simulink model "Tactical_ACC_trainlm_3_15_Jan_5"  (R2021a)
settings: Solver=FixedStepAuto  StartTime=0.0  StopTime=T  FixedStep=Ts  RelTol=1e-3
undefined symbols (not defined in the file): Ts, v0_ego, v0_lead, x0_ego, x0_lead
libraries: neural x50
(part 2 of 2)

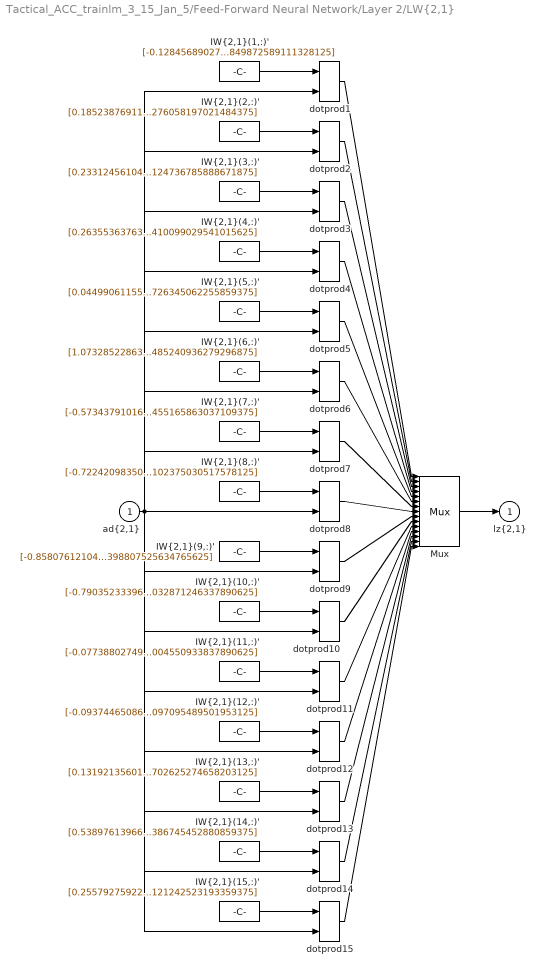
== system Tactical_ACC_trainlm_3_15_Jan_5/Feed-Forward Neural Network/Layer 2/LW{2,1} ==
  "ad{2,1}" : Inport  PortDimensions=15
      mask Display: e = 0.06;c1 = [120 230 180]/255;c2 = ([120 230 180]+0)/(256+128);c3 = ([120 230 180]+128)/(256+128);patch([0 1 1 0],[0 0 1 1],c1);patch([0 1 1 1-e 1-e 0+e],[0 0 1 1-e 0+e 0+e],c2);patch([0 0 1 1-e 0+e 0+e],[0 1 1 1-e 1-e 0+e],c3);plot([0 1 1 0 0],[0 0 1 1 0]);
  "IW{2,1}(1,:)'" : Constant  Value=[-0.1284568902708948245905418161783018149435520172119140625;0.54389311937212003744690491657820530235767364501953125;0.53673915075766809312796112862997688353061676025390625;-0.96084475289336257475270031136460602283477783203125;-0.39150449404426834743020435780636034905910491943359375;-0.1860903257221864226522711760480888187885284423828125;0.7272658289096070038937114077270962297916412353515625;-0.54431412858791627940036050858907401561737060546875;0.5380581706717924017624454791075550019741058349609375;-0.9009348419158775822523921306128613650798797607421875;-0.402444399393438401180134178503067232668399810791015625;-0.5338710106559780843582529996638186275959014892578125;-0.83906258199989902646365180771681480109691619873046875;-0.64876603531735022034609983165864832699298858642578125;0.179996379296625708121837305952794849872589111328125]
      mask Display: e = 0.06;c1 = [120 150 230]/255;c2 = ([120 150 230]+0)/383;c3 = ([120 150 230]+128)/383;patch([0 1 1 0],[0 0 1 1],c1);patch([0 1 1 1-e 1-e 0+e],[0 0 1 1-e 0+e 0+e],c2);patch([0 0 1 1-e 0+e 0+e],[0 1 1 1-e 1-e 0+e],c3);plot([0 1 1 0 0],[0 0 1 1 0]);disp('weights');
  "IW{2,1}(10,:)'" : Constant  Value=[-0.79035233396170545550063479822711087763309478759765625;0.72237775299588691257923755983938463032245635986328125;-0.306611429735239748861630459941807202994823455810546875;0.5382287747765912566677570794126950204372406005859375;0.99699154938168776940443649436929263174533843994140625;0.3573046096003764660054002888500690460205078125;0.59913861015160729817097262639435939490795135498046875;-0.8330343727947546739187600906006991863250732421875;-0.581189831958130564970588238793425261974334716796875;-0.4362662882391401542037101535242982208728790283203125;-0.382792034697409022658831645458121784031391143798828125;1.4688049411392551935051642431062646210193634033203125;0.79640769268750644105381297777057625353336334228515625;-0.4162072596359613907424090939457528293132781982421875;-0.181387517948383314436711089001619257032871246337890625]
      mask Display: e = 0.06;c1 = [120 150 230]/255;c2 = ([120 150 230]+0)/383;c3 = ([120 150 230]+128)/383;patch([0 1 1 0],[0 0 1 1],c1);patch([0 1 1 1-e 1-e 0+e],[0 0 1 1-e 0+e 0+e],c2);patch([0 0 1 1-e 0+e 0+e],[0 1 1 1-e 1-e 0+e],c3);plot([0 1 1 0 0],[0 0 1 1 0]);disp('weights');
  "IW{2,1}(11,:)'" : Constant  Value=[-0.07738802749405981895591821739799343049526214599609375;-0.030300753448414353974360579968561069108545780181884765625;0.13159391893646643634241399922757409512996673583984375;-0.2064169659727668193482941205729730427265167236328125;0.042509571957955911980509000613892567344009876251220703125;-0.0096459618206787833827320355339907109737396240234375;0.374231149766926451949444754063733853399753570556640625;0.25191957034316647678906520013697445392608642578125;0.1045826830775500315695580866304226219654083251953125;0.07719335609068078696282100281678140163421630859375;0.635756796826290493385158697492443025112152099609375;0.10699981116102953715429890735322260297834873199462890625;-0.152211268792612097744409993538283742964267730712890625;-0.164472335625503174316719423586619086563587188720703125;0.79116563379986681869837639169418253004550933837890625]
      mask Display: e = 0.06;c1 = [120 150 230]/255;c2 = ([120 150 230]+0)/383;c3 = ([120 150 230]+128)/383;patch([0 1 1 0],[0 0 1 1],c1);patch([0 1 1 1-e 1-e 0+e],[0 0 1 1-e 0+e 0+e],c2);patch([0 0 1 1-e 0+e 0+e],[0 1 1 1-e 1-e 0+e],c3);plot([0 1 1 0 0],[0 0 1 1 0]);disp('weights');
  "IW{2,1}(12,:)'" : Constant  Value=[-0.09374465086869930574575704440576373599469661712646484375;-0.21310105235882270680036754129105247557163238525390625;-0.10868460812037449014777479305848828516900539398193359375;0.617028191774690260018587650847621262073516845703125;0.77303193361052124910060001639067195355892181396484375;-0.6205791879648396847102276296936906874179840087890625;0.92080509229272256011000763464835472404956817626953125;0.32188911589468460761054302565753459930419921875;0.25976677012884241690926501178182661533355712890625;0.390326078888663996480090645491145551204681396484375;-0.6818652671110874141646718271658755838871002197265625;0.8765389199457593871755989312077872455120086669921875;0.85347912612335619098047345687518827617168426513671875;-0.057448392693464189751040294140693731606006622314453125;-0.7914071094984909127134642403689213097095489501953125]
      mask Display: e = 0.06;c1 = [120 150 230]/255;c2 = ([120 150 230]+0)/383;c3 = ([120 150 230]+128)/383;patch([0 1 1 0],[0 0 1 1],c1);patch([0 1 1 1-e 1-e 0+e],[0 0 1 1-e 0+e 0+e],c2);patch([0 0 1 1-e 0+e 0+e],[0 1 1 1-e 1-e 0+e],c3);plot([0 1 1 0 0],[0 0 1 1 0]);disp('weights');
  "IW{2,1}(13,:)'" : Constant  Value=[0.1319213560109291638600126361779985018074512481689453125;0.342914070048148500458040643934509716928005218505859375;0.17346245905404111820047319270088337361812591552734375;0.5101541980141670595827463330351747572422027587890625;0.2116092910741979860045347550112637691199779510498046875;-0.0099883500195583341252358877682127058506011962890625;0.07323493448403718686368080170723260380327701568603515625;0.459503710634442175120284446165896952152252197265625;-0.9360179684748661799176261411048471927642822265625;-0.0017679730348210132007125139352865517139434814453125;-0.78093606800248605015468683632207103073596954345703125;-0.165663696750330158291575344264856539666652679443359375;-0.26863726210748828382435249295667745172977447509765625;0.443776146337074350878282302801380865275859832763671875;0.475654128018537403210785896590095944702625274658203125]
      mask Display: e = 0.06;c1 = [120 150 230]/255;c2 = ([120 150 230]+0)/383;c3 = ([120 150 230]+128)/383;patch([0 1 1 0],[0 0 1 1],c1);patch([0 1 1 1-e 1-e 0+e],[0 0 1 1-e 0+e 0+e],c2);patch([0 0 1 1-e 0+e 0+e],[0 1 1 1-e 1-e 0+e],c3);plot([0 1 1 0 0],[0 0 1 1 0]);disp('weights');
  "IW{2,1}(14,:)'" : Constant  Value=[0.5389761396637500201478587769088335335254669189453125;0.48251476910261115182976254800450988113880157470703125;0.57826646044851981454115730230114422738552093505859375;-0.2452089103297943051273932724143378436565399169921875;-1.179601056993847318921098121791146695613861083984375;-0.7047835560466226834108738330542109906673431396484375;-0.1688329075373741494647816807628259994089603424072265625;0.78150423265064450362160641816444694995880126953125;0.2294268382342810053131643144297413527965545654296875;0.071602111502226506445367704145610332489013671875;-0.5583507712921489396507013225345872342586517333984375;-1.040588019370590533441145453252829611301422119140625;-0.417402993887157902630491435047588311135768890380859375;0.6362951341913660741056446568109095096588134765625;0.837706070944830738511654999456368386745452880859375]
      mask Display: e = 0.06;c1 = [120 150 230]/255;c2 = ([120 150 230]+0)/383;c3 = ([120 150 230]+128)/383;patch([0 1 1 0],[0 0 1 1],c1);patch([0 1 1 1-e 1-e 0+e],[0 0 1 1-e 0+e 0+e],c2);patch([0 0 1 1-e 0+e 0+e],[0 1 1 1-e 1-e 0+e],c3);plot([0 1 1 0 0],[0 0 1 1 0]);disp('weights');
  "IW{2,1}(15,:)'" : Constant  Value=[0.25579275922833755174679026822559535503387451171875;0.040104934780773593416824951418675482273101806640625;-0.11538917323325836861158677493222057819366455078125;-0.56796216807721133790209933067671954631805419921875;-0.6002743542850959013179590328945778310298919677734375;-0.890051706187623636878925026394426822662353515625;0.6026952110439045551260051070130430161952972412109375;0.964606445767212772324228353681974112987518310546875;-0.2751770754538946928136056158109568059444427490234375;-0.10963366940791541281896570581011474132537841796875;-0.667079118247158486809667010675184428691864013671875;-0.2028210065283138074931912342435680329799652099609375;-0.891521031117740836435814344440586864948272705078125;-0.799556919609016869543438588152639567852020263671875;0.12372285056327481100879595032893121242523193359375]
      mask Display: e = 0.06;c1 = [120 150 230]/255;c2 = ([120 150 230]+0)/383;c3 = ([120 150 230]+128)/383;patch([0 1 1 0],[0 0 1 1],c1);patch([0 1 1 1-e 1-e 0+e],[0 0 1 1-e 0+e 0+e],c2);patch([0 0 1 1-e 0+e 0+e],[0 1 1 1-e 1-e 0+e],c3);plot([0 1 1 0 0],[0 0 1 1 0]);disp('weights');
  "IW{2,1}(2,:)'" : Constant  Value=[0.185238769116202905973267434092122130095958709716796875;0.86572745162572328769812202153843827545642852783203125;-0.5993331590168649025684999287477694451808929443359375;-0.3382842395718579364682909726980142295360565185546875;0.92854655533397656430594224730157293379306793212890625;0.4974114364313828584585053249611519277095794677734375;0.08349591760344533819537815588773810304701328277587890625;-0.003811417607220590753058786503970623016357421875;0.162892975750795532263737186440266668796539306640625;-0.0208600216453564968333012075163424015045166015625;0.09994084869043064200955228670864016748964786529541015625;0.6505716295410695071410600576200522482395172119140625;-0.74344937140645417361639601949718780815601348876953125;0.311377290880280488405418282127357088029384613037109375;-0.370413344649913101047644659047364257276058197021484375]
      mask Display: e = 0.06;c1 = [120 150 230]/255;c2 = ([120 150 230]+0)/383;c3 = ([120 150 230]+128)/383;patch([0 1 1 0],[0 0 1 1],c1);patch([0 1 1 1-e 1-e 0+e],[0 0 1 1-e 0+e 0+e],c2);patch([0 0 1 1-e 0+e 0+e],[0 1 1 1-e 1-e 0+e],c3);plot([0 1 1 0 0],[0 0 1 1 0]);disp('weights');
  "IW{2,1}(3,:)'" : Constant  Value=[0.2331245610411065982692235820650239475071430206298828125;0.94534056286266598956302686929120682179927825927734375;0.73477219805281890341319694925914518535137176513671875;-0.1513810063337250877424366990453563630580902099609375;-1.2712555974780930245771060072002001106739044189453125;0.6511676315723111674316214703139849007129669189453125;0.8116798971944201301909060930483974516391754150390625;0.801704977064009671750000052270479500293731689453125;0.856626124628375951175485170097090303897857666015625;-0.6149792078758504754176783535513095557689666748046875;0.9912444394374702039129942932049743831157684326171875;-1.6174591172065169164540066049084998667240142822265625;0.7343427724308513315776281160651706159114837646484375;-0.373115221066490587720210214683902449905872344970703125;-0.307431976628442071852731487524579279124736785888671875]
      mask Display: e = 0.06;c1 = [120 150 230]/255;c2 = ([120 150 230]+0)/383;c3 = ([120 150 230]+128)/383;patch([0 1 1 0],[0 0 1 1],c1);patch([0 1 1 1-e 1-e 0+e],[0 0 1 1-e 0+e 0+e],c2);patch([0 0 1 1-e 0+e 0+e],[0 1 1 1-e 1-e 0+e],c3);plot([0 1 1 0 0],[0 0 1 1 0]);disp('weights');
  "IW{2,1}(4,:)'" : Constant  Value=[0.26355363763175121416537649565725587308406829833984375;-0.6159994507456831858149826075532473623752593994140625;-0.309763994465098335684416497315396554768085479736328125;-0.4594591531358693803355208729044534265995025634765625;0.366643413083722002898667824410949833691120147705078125;0.579926059889061651375641304184682667255401611328125;0.496490583582257893890954392190906219184398651123046875;0.1493224382603752786735640256665647029876708984375;0.1601807315168832790419628508971072733402252197265625;-0.753832504908109601871046834276057779788970947265625;0.66482363338864047808129953409661538898944854736328125;0.7047628961209226883255496431956999003887176513671875;-0.597867900421577669334283200441859662532806396484375;0.84600607163113539233023630004026927053928375244140625;0.1183481655249266906171357049970538355410099029541015625]
      mask Display: e = 0.06;c1 = [120 150 230]/255;c2 = ([120 150 230]+0)/383;c3 = ([120 150 230]+128)/383;patch([0 1 1 0],[0 0 1 1],c1);patch([0 1 1 1-e 1-e 0+e],[0 0 1 1-e 0+e 0+e],c2);patch([0 0 1 1-e 0+e 0+e],[0 1 1 1-e 1-e 0+e],c3);plot([0 1 1 0 0],[0 0 1 1 0]);disp('weights');
  "IW{2,1}(5,:)'" : Constant  Value=[0.0449906115542042517319032413070090115070343017578125;-0.7222515943416893957618185595492832362651824951171875;-0.9110918154435230231769082820392213761806488037109375;-0.6058924038090884867102658972726203501224517822265625;-0.122710034826088776327424056944437325000762939453125;-0.3629515092020156874497160970349796116352081298828125;0.165581930351680117752266596653498709201812744140625;0.6903563701080732695203323601162992417812347412109375;-0.96603412332547744512112330994568765163421630859375;-0.5890116581846402965538800344802439212799072265625;-0.45941133541460477118789640371687710285186767578125;0.457323363356542333946208600536920130252838134765625;-0.408932331049287167701322687207721173763275146484375;-0.763689603106578740465693044825457036495208740234375;-0.3283020506461509224749306667945347726345062255859375]
      mask Display: e = 0.06;c1 = [120 150 230]/255;c2 = ([120 150 230]+0)/383;c3 = ([120 150 230]+128)/383;patch([0 1 1 0],[0 0 1 1],c1);patch([0 1 1 1-e 1-e 0+e],[0 0 1 1-e 0+e 0+e],c2);patch([0 0 1 1-e 0+e 0+e],[0 1 1 1-e 1-e 0+e],c3);plot([0 1 1 0 0],[0 0 1 1 0]);disp('weights');
  "IW{2,1}(6,:)'" : Constant  Value=[1.073285228639864641309031867422163486480712890625;0.392495340995861308197589778501424007117748260498046875;0.4850650961144948869474546881974674761295318603515625;0.6434423699226197168599128417554311454296112060546875;0.680041364342549581323282836819998919963836669921875;0.0681282547414527872575717992731370031833648681640625;0.64862678540349472111614659297629259526729583740234375;0.47728058399080364182509583770297467708587646484375;-0.7582808578028836787865429869270883500576019287109375;-0.7069701787702202810947937905439175665378570556640625;-0.6662159570437304889622964765294454991817474365234375;0.1711366707004692566673753617578768171370029449462890625;-0.346231314906966514133301870970171876251697540283203125;0.9654623989469779399286153420689515769481658935546875;-0.60325600334875761898700829988229088485240936279296875]
      mask Display: e = 0.06;c1 = [120 150 230]/255;c2 = ([120 150 230]+0)/383;c3 = ([120 150 230]+128)/383;patch([0 1 1 0],[0 0 1 1],c1);patch([0 1 1 1-e 1-e 0+e],[0 0 1 1-e 0+e 0+e],c2);patch([0 0 1 1-e 0+e 0+e],[0 1 1 1-e 1-e 0+e],c3);plot([0 1 1 0 0],[0 0 1 1 0]);disp('weights');
  "IW{2,1}(7,:)'" : Constant  Value=[-0.57343791016769840584998974009067751467227935791015625;-0.81230175846522756355483352308510802686214447021484375;-0.460163965563413768222744693048298358917236328125;-0.140157181233467209580112466937862336635589599609375;0.595545978896323102702581309131346642971038818359375;-0.82009864245883790090374532155692577362060546875;0.7869613238475354766165992259630002081394195556640625;0.17197407165295164332974309218116104602813720703125;0.725421437399339286145050209597684442996978759765625;-0.621855651054772362584799338947050273418426513671875;0.129854351950570212625990507149253971874713897705078125;-0.85541353023072674854887509354739449918270111083984375;-0.066954344696821710414269546163268387317657470703125;0.08686990560648304160462629397443379275500774383544921875;-0.56968257593998483656605458236299455165863037109375]
      mask Display: e = 0.06;c1 = [120 150 230]/255;c2 = ([120 150 230]+0)/383;c3 = ([120 150 230]+128)/383;patch([0 1 1 0],[0 0 1 1],c1);patch([0 1 1 1-e 1-e 0+e],[0 0 1 1-e 0+e 0+e],c2);patch([0 0 1 1-e 0+e 0+e],[0 1 1 1-e 1-e 0+e],c3);plot([0 1 1 0 0],[0 0 1 1 0]);disp('weights');
  "IW{2,1}(8,:)'" : Constant  Value=[-0.7224209835068311491568238125182688236236572265625;0.050869593250156990016375146979044075123965740203857421875;0.21859062205123958033681219603749923408031463623046875;0.7755419085127075451424616403528489172458648681640625;-0.98730531091106688013070424858597107231616973876953125;-0.776588511613593102111963162315078079700469970703125;0.792481707072821617288127526990137994289398193359375;-0.5065309480280502096860573146841488778591156005859375;-0.031406977575795025359184364788234233856201171875;-0.9146951781777132861606105507235042750835418701171875;0.49203673068935105394672291367896832525730133056640625;0.41480058077774961677874898668960668146610260009765625;0.183304582750635047805332078496576286852359771728515625;0.385143116164009813306989826742210425436496734619140625;1.1302421062639844695496549320523627102375030517578125]
      mask Display: e = 0.06;c1 = [120 150 230]/255;c2 = ([120 150 230]+0)/383;c3 = ([120 150 230]+128)/383;patch([0 1 1 0],[0 0 1 1],c1);patch([0 1 1 1-e 1-e 0+e],[0 0 1 1-e 0+e 0+e],c2);patch([0 0 1 1-e 0+e 0+e],[0 1 1 1-e 1-e 0+e],c3);plot([0 1 1 0 0],[0 0 1 1 0]);disp('weights');
  "IW{2,1}(9,:)'" : Constant  Value=[-0.85807612104994845925176605305750854313373565673828125;0.060642466524505611591422393757966347038745880126953125;0.67053556318306017924868456248077563941478729248046875;-0.2176340090776733848798585313488729298114776611328125;0.498101819152965752390826992268557660281658172607421875;-0.727414902123402651312744637834839522838592529296875;-1.0967891667210161177337113258545286953449249267578125;0.3328324346389359700282284393324516713619232177734375;0.6897113491525264095116654061712324619293212890625;0.270395833719764056013445951975882053375244140625;-0.1297060102155986049954350391999469138681888580322265625;0.62727037435593546721435131985344924032688140869140625;-0.9040101576978389896765975208836607635021209716796875;1.003263748472904115516257661511190235614776611328125;0.541537544987497287962696645990945398807525634765625]
      mask Display: e = 0.06;c1 = [120 150 230]/255;c2 = ([120 150 230]+0)/383;c3 = ([120 150 230]+128)/383;patch([0 1 1 0],[0 0 1 1],c1);patch([0 1 1 1-e 1-e 0+e],[0 0 1 1-e 0+e 0+e],c2);patch([0 0 1 1-e 0+e 0+e],[0 1 1 1-e 1-e 0+e],c3);plot([0 1 1 0 0],[0 0 1 1 0]);disp('weights');
  Mux : Mux  Inputs=15
      mask Display: e = 0.06;c1 = [120 150 230]/255;c2 = ([120 150 230]+0)/383;c3 = ([120 150 230]+128)/383;patch([0 1 1 0],[0 0 1 1],c1);patch([0 1 1 1-e 1-e 0+e],[0 0 1 1-e 0+e 0+e],c2);patch([0 0 1 1-e 0+e 0+e],[0 1 1 1-e 1-e 0+e],c3);plot([0 1 1 0 0],[0 0 1 1 0]);disp('Mux');
  dotprod{1..15} (15 alike) : neural/Weight Functions/dotprod
  "lz{2,1}" : Outport
      mask Display: e = 0.06;c1 = [120 230 180]/255;c2 = ([120 230 180]+0)/(256+128);c3 = ([120 230 180]+128)/(256+128);patch([0 1 1 0],[0 0 1 1],c1);patch([0 1 1 1-e 1-e 0+e],[0 0 1 1-e 0+e 0+e],c2);patch([0 0 1 1-e 0+e 0+e],[0 1 1 1-e 1-e 0+e],c3);plot([0 1 1 0 0],[0 0 1 1 0]);
  wires:
  "IW{2,1}(1,:)'"/1 -> dotprod1/1
  "ad{2,1}"/1 -> dotprod1/2, dotprod2/2, dotprod3/2, dotprod4/2, dotprod5/2, dotprod6/2, dotprod7/2, dotprod8/2, dotprod9/2, dotprod10/2, dotprod11/2, dotprod12/2, dotprod13/2, dotprod14/2, dotprod15/2
  dotprod1/1 -> Mux/1
  "IW{2,1}(2,:)'"/1 -> dotprod2/1
  dotprod2/1 -> Mux/2
  "IW{2,1}(3,:)'"/1 -> dotprod3/1
  dotprod3/1 -> Mux/3
  "IW{2,1}(4,:)'"/1 -> dotprod4/1
  dotprod4/1 -> Mux/4
  "IW{2,1}(5,:)'"/1 -> dotprod5/1
  dotprod5/1 -> Mux/5
  "IW{2,1}(6,:)'"/1 -> dotprod6/1
  dotprod6/1 -> Mux/6
  "IW{2,1}(7,:)'"/1 -> dotprod7/1
  dotprod7/1 -> Mux/7
  "IW{2,1}(8,:)'"/1 -> dotprod8/1
  dotprod8/1 -> Mux/8
  "IW{2,1}(9,:)'"/1 -> dotprod9/1
  dotprod9/1 -> Mux/9
  "IW{2,1}(10,:)'"/1 -> dotprod10/1
  dotprod10/1 -> Mux/10
  "IW{2,1}(11,:)'"/1 -> dotprod11/1
  dotprod11/1 -> Mux/11
  "IW{2,1}(12,:)'"/1 -> dotprod12/1
  dotprod12/1 -> Mux/12
  "IW{2,1}(13,:)'"/1 -> dotprod13/1
  dotprod13/1 -> Mux/13
  "IW{2,1}(14,:)'"/1 -> dotprod14/1
  dotprod14/1 -> Mux/14
  "IW{2,1}(15,:)'"/1 -> dotprod15/1
  dotprod15/1 -> Mux/15
  Mux/1 -> "lz{2,1}"/1

== system Tactical_ACC_trainlm_3_15_Jan_5/Feed-Forward Neural Network/Layer 3/Delays 1 ==
  "p{3}" : Inport  PortDimensions=15
      mask Display: e = 0.06;c1 = [120 230 180]/255;c2 = ([120 230 180]+0)/(256+128);c3 = ([120 230 180]+128)/(256+128);patch([0 1 1 0],[0 0 1 1],c1);patch([0 1 1 1-e 1-e 0+e],[0 0 1 1-e 0+e 0+e],c2);patch([0 0 1 1-e 0+e 0+e],[0 1 1 1-e 1-e 0+e],c3);plot([0 1 1 0 0],[0 0 1 1 0]);
  mux : Mux  Inputs=1
      mask Display: e = 0.06;c1 = [120 150 230]/255;c2 = ([120 150 230]+0)/383;c3 = ([120 150 230]+128)/383;patch([0 1 1 0],[0 0 1 1],c1);patch([0 1 1 1-e 1-e 0+e],[0 0 1 1-e 0+e 0+e],c2);patch([0 0 1 1-e 0+e 0+e],[0 1 1 1-e 1-e 0+e],c3);plot([0 1 1 0 0],[0 0 1 1 0]);disp('Mux')
  "pd{3,2}" : Outport
      mask Display: e = 0.06;c1 = [120 230 180]/255;c2 = ([120 230 180]+0)/(256+128);c3 = ([120 230 180]+128)/(256+128);patch([0 1 1 0],[0 0 1 1],c1);patch([0 1 1 1-e 1-e 0+e],[0 0 1 1-e 0+e 0+e],c2);patch([0 0 1 1-e 0+e 0+e],[0 1 1 1-e 1-e 0+e],c3);plot([0 1 1 0 0],[0 0 1 1 0]);
  wires:
  "p{3}"/1 -> mux/1
  mux/1 -> "pd{3,2}"/1

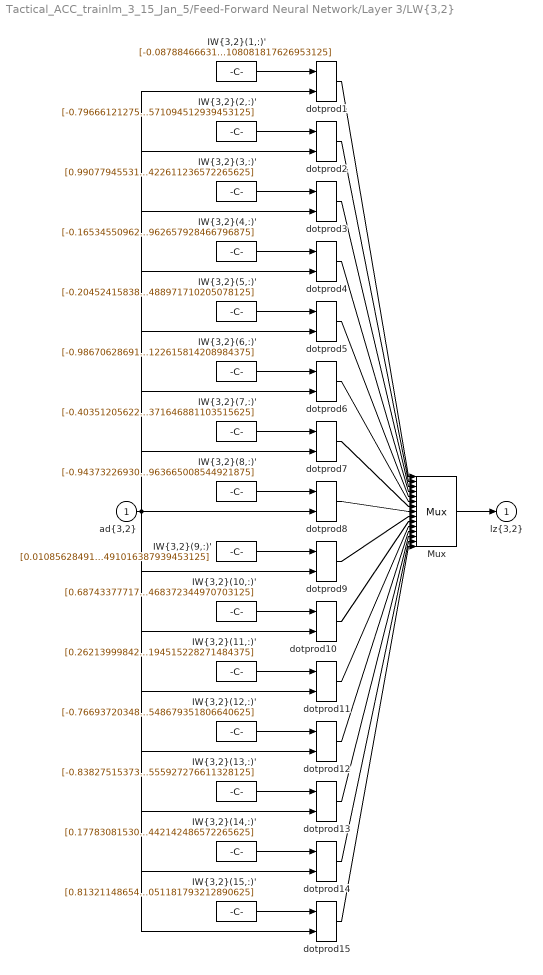
== system Tactical_ACC_trainlm_3_15_Jan_5/Feed-Forward Neural Network/Layer 3/LW{3,2} ==
  "ad{3,2}" : Inport  PortDimensions=15
      mask Display: e = 0.06;c1 = [120 230 180]/255;c2 = ([120 230 180]+0)/(256+128);c3 = ([120 230 180]+128)/(256+128);patch([0 1 1 0],[0 0 1 1],c1);patch([0 1 1 1-e 1-e 0+e],[0 0 1 1-e 0+e 0+e],c2);patch([0 0 1 1-e 0+e 0+e],[0 1 1 1-e 1-e 0+e],c3);plot([0 1 1 0 0],[0 0 1 1 0]);
  "IW{3,2}(1,:)'" : Constant  Value=[-0.0878846663125170124430951545946300029754638671875;0.0675439035340004156893201070488430559635162353515625;0.3850639727730376105085952076478861272335052490234375;-0.897336227775257899708094555535353720188140869140625;0.4800646559755552544856982422061264514923095703125;-0.5886509570704803184781894742627628147602081298828125;-0.7754320756879466980393544872640632092952728271484375;-0.0247924491321527273868241536547429859638214111328125;-0.81529532256159686909313677460886538028717041015625;-0.367142001707418064171406513196416199207305908203125;0.9758694699049907939070180873386561870574951171875;-0.2984465102282147785928145822254009544849395751953125;-0.750254482560374302835271009826101362705230712890625;-0.07347884281256167327001094236038625240325927734375;0.61840770258758670507859278586693108081817626953125]
      mask Display: e = 0.06;c1 = [120 150 230]/255;c2 = ([120 150 230]+0)/383;c3 = ([120 150 230]+128)/383;patch([0 1 1 0],[0 0 1 1],c1);patch([0 1 1 1-e 1-e 0+e],[0 0 1 1-e 0+e 0+e],c2);patch([0 0 1 1-e 0+e 0+e],[0 1 1 1-e 1-e 0+e],c3);plot([0 1 1 0 0],[0 0 1 1 0]);disp('weights');
  "IW{3,2}(10,:)'" : Constant  Value=[0.68743377717876719135148277928237803280353546142578125;0.0164115705993483247671083091745458659715950489044189453125;-0.7366864626889284561883641799795441329479217529296875;-0.2545087325302743952448736308724619448184967041015625;0.1958832707677782281052714097313582897186279296875;-0.389178760778625398852881289712968282401561737060546875;0.298243617485746737028051711604348383843898773193359375;0.011473260083985629964598018659671652130782604217529296875;-0.8168763302649721946835370545159094035625457763671875;1.082137349653022884155006977380253374576568603515625;-0.1494947230984948749465957007487304508686065673828125;0.167419649068595910446077823507948778569698333740234375;0.262483437056319157676398390321992337703704833984375;-1.6514659181993354142292673714109696447849273681640625;-0.489226519023898465121646950137801468372344970703125]
      mask Display: e = 0.06;c1 = [120 150 230]/255;c2 = ([120 150 230]+0)/383;c3 = ([120 150 230]+128)/383;patch([0 1 1 0],[0 0 1 1],c1);patch([0 1 1 1-e 1-e 0+e],[0 0 1 1-e 0+e 0+e],c2);patch([0 0 1 1-e 0+e 0+e],[0 1 1 1-e 1-e 0+e],c3);plot([0 1 1 0 0],[0 0 1 1 0]);disp('weights');
  "IW{3,2}(11,:)'" : Constant  Value=[0.262139998427187048690711890230886638164520263671875;0.0522049315911223832387122456566430628299713134765625;0.0990802140303959077982653980143368244171142578125;0.2814358459318511140878626974881626665592193603515625;0.5787278872838108600973328066174872219562530517578125;-0.5252539605888415508161415345966815948486328125;-0.780489898553896832567033925442956387996673583984375;-0.3683771233222679075680616733734495937824249267578125;-0.8028118145780045455950357791152782738208770751953125;0.4134304353938611509278189259930513799190521240234375;-0.691260389041455258762880475842393934726715087890625;-0.2807873640555287320097477277158759534358978271484375;0.518654766262192534753694417304359376430511474609375;-0.692819246761199547535170495393685996532440185546875;-0.9589284506836308619170949896215461194515228271484375]
      mask Display: e = 0.06;c1 = [120 150 230]/255;c2 = ([120 150 230]+0)/383;c3 = ([120 150 230]+128)/383;patch([0 1 1 0],[0 0 1 1],c1);patch([0 1 1 1-e 1-e 0+e],[0 0 1 1-e 0+e 0+e],c2);patch([0 0 1 1-e 0+e 0+e],[0 1 1 1-e 1-e 0+e],c3);plot([0 1 1 0 0],[0 0 1 1 0]);disp('weights');
  "IW{3,2}(12,:)'" : Constant  Value=[-0.76693720348648930507096110886777751147747039794921875;0.5481856490673935322632814859389327466487884521484375;-0.0173256676970391411407579340675511048175394535064697265625;-0.2227443390360405450767444790471927262842655181884765625;-0.26469416312424609571962719201110303401947021484375;0.1327473606630025226849056707578711211681365966796875;0.880155040053234305474916254752315580844879150390625;0.9313590226680583672447255594306625425815582275390625;-0.6076771681973791583430966056766919791698455810546875;0.164603200714055597497775806914432905614376068115234375;-0.1916974103070070156729087784697185270488262176513671875;0.149175496388683825887966349910129792988300323486328125;0.4442873994484541899652185747982002794742584228515625;0.60908523871015962658503894999739713966846466064453125;0.8473512252408144096449404969462193548679351806640625]
      mask Display: e = 0.06;c1 = [120 150 230]/255;c2 = ([120 150 230]+0)/383;c3 = ([120 150 230]+128)/383;patch([0 1 1 0],[0 0 1 1],c1);patch([0 1 1 1-e 1-e 0+e],[0 0 1 1-e 0+e 0+e],c2);patch([0 0 1 1-e 0+e 0+e],[0 1 1 1-e 1-e 0+e],c3);plot([0 1 1 0 0],[0 0 1 1 0]);disp('weights');
  "IW{3,2}(13,:)'" : Constant  Value=[-0.8382751537393726692926065879873931407928466796875;0.414506970630843074587801311281509697437286376953125;0.7809513583688765248069785229745320975780487060546875;0.3076240451915472906563309152261354029178619384765625;-0.5879442809896107124956188272335566580295562744140625;-0.81700253732117555927061403053812682628631591796875;-0.62507838715662700224129366688430309295654296875;0.3928659780121896982763018968398682773113250732421875;-0.6634974030169444869642347839544527232646942138671875;-0.3731420201268174086095541497343219816684722900390625;-0.6777320563012783072309730414417572319507598876953125;0.4850907314038781503739983236300759017467498779296875;0.4873766829746519757549094720161519944667816162109375;0.0817681624829529329900879019987769424915313720703125;0.3073997780165058646417719501187093555927276611328125]
      mask Display: e = 0.06;c1 = [120 150 230]/255;c2 = ([120 150 230]+0)/383;c3 = ([120 150 230]+128)/383;patch([0 1 1 0],[0 0 1 1],c1);patch([0 1 1 1-e 1-e 0+e],[0 0 1 1-e 0+e 0+e],c2);patch([0 0 1 1-e 0+e 0+e],[0 1 1 1-e 1-e 0+e],c3);plot([0 1 1 0 0],[0 0 1 1 0]);disp('weights');
  "IW{3,2}(14,:)'" : Constant  Value=[0.1778308153014782899692391993085038848221302032470703125;0.52463729139749737395703732545371167361736297607421875;2.230250057260251939084128025569953024387359619140625;0.5030503612490930809286737712682224810123443603515625;-0.8266669052089354874368609671364538371562957763671875;0.06677773512409916623067118734979885630309581756591796875;-0.412912205520802710889682884953799657523632049560546875;0.1054167204125333601183456266880966722965240478515625;-0.414603408605299705858016068305005319416522979736328125;-0.466950678721560652473243635540711693465709686279296875;0.242839314268684436370904222712852060794830322265625;0.2177309558120963384197921186569146811962127685546875;-0.84248454167226938249513068512897007167339324951171875;-1.3537046097364704433374527070554904639720916748046875;0.8652271440971281979415152818546630442142486572265625]
      mask Display: e = 0.06;c1 = [120 150 230]/255;c2 = ([120 150 230]+0)/383;c3 = ([120 150 230]+128)/383;patch([0 1 1 0],[0 0 1 1],c1);patch([0 1 1 1-e 1-e 0+e],[0 0 1 1-e 0+e 0+e],c2);patch([0 0 1 1-e 0+e 0+e],[0 1 1 1-e 1-e 0+e],c3);plot([0 1 1 0 0],[0 0 1 1 0]);disp('weights');
  "IW{3,2}(15,:)'" : Constant  Value=[0.813211486545263095848667944665066897869110107421875;-0.419622632984383681087336981363478116691112518310546875;0.46867819330040705327888872488983906805515289306640625;0.1694393821494001028948872544788173399865627288818359375;0.543867834198214605834209578461013734340667724609375;-0.790158192045417262505679900641553103923797607421875;0.5953226747136171059793241511215455830097198486328125;-0.73861776286557379034292125652427785098552703857421875;-0.364510165293153942656090293894521892070770263671875;0.23663618486601922796808139537461102008819580078125;0.7389557671922355464033671523793600499629974365234375;-0.1465994822378131612339302591863088309764862060546875;0.363005995666967173907124788456712849438190460205078125;-0.92498077594266892020868908730335533618927001953125;-0.6729752629449488043889004984521307051181793212890625]
      mask Display: e = 0.06;c1 = [120 150 230]/255;c2 = ([120 150 230]+0)/383;c3 = ([120 150 230]+128)/383;patch([0 1 1 0],[0 0 1 1],c1);patch([0 1 1 1-e 1-e 0+e],[0 0 1 1-e 0+e 0+e],c2);patch([0 0 1 1-e 0+e 0+e],[0 1 1 1-e 1-e 0+e],c3);plot([0 1 1 0 0],[0 0 1 1 0]);disp('weights');
  "IW{3,2}(2,:)'" : Constant  Value=[-0.7966612127504897333807321047061122953891754150390625;-0.7816915759150828701962154809734784066677093505859375;0.1133396699280251329611246546846814453601837158203125;-0.854229401802047760838831891305744647979736328125;-0.530346170504191416483763532596640288829803466796875;-0.2234567379043965740237354111741296947002410888671875;0.5688557814878254514923128226655535399913787841796875;0.5379165281177382684774102017399854958057403564453125;-0.9843594128613302185470956828794442117214202880859375;-0.564873381154358700229067835607565939426422119140625;-0.6591359538862333611319854753674007952213287353515625;0.3710714174950744403957969552720896899700164794921875;-0.951131967899252028786349910660646855831146240234375;-0.5756735894901312544646998503594659268856048583984375;0.4972377435523942512674011595663614571094512939453125]
      mask Display: e = 0.06;c1 = [120 150 230]/255;c2 = ([120 150 230]+0)/383;c3 = ([120 150 230]+128)/383;patch([0 1 1 0],[0 0 1 1],c1);patch([0 1 1 1-e 1-e 0+e],[0 0 1 1-e 0+e 0+e],c2);patch([0 0 1 1-e 0+e 0+e],[0 1 1 1-e 1-e 0+e],c3);plot([0 1 1 0 0],[0 0 1 1 0]);disp('weights');
  "IW{3,2}(3,:)'" : Constant  Value=[0.9907794553101834100772293822956271469593048095703125;0.6516177157111966433689076438895426690578460693359375;-0.20695841483681487460444259340874850749969482421875;-0.8229450806505591575756852762424387037754058837890625;0.4699150833921044156937796287820674479007720947265625;0.103557063914454960951161410775966942310333251953125;-0.416859364186138225960576164652593433856964111328125;-0.2079865095642496886085837104474194347858428955078125;-0.1537812296716669635543439653702080249786376953125;-0.4979163079685278159303152278880588710308074951171875;-0.4844154988559739027920159060158766806125640869140625;-0.4117027324643007801796557032503187656402587890625;-0.4196294697385456462512820507981814444065093994140625;-0.8029625246237832580931126358336769044399261474609375;-0.7596259640258387069167156369076110422611236572265625]
      mask Display: e = 0.06;c1 = [120 150 230]/255;c2 = ([120 150 230]+0)/383;c3 = ([120 150 230]+128)/383;patch([0 1 1 0],[0 0 1 1],c1);patch([0 1 1 1-e 1-e 0+e],[0 0 1 1-e 0+e 0+e],c2);patch([0 0 1 1-e 0+e 0+e],[0 1 1 1-e 1-e 0+e],c3);plot([0 1 1 0 0],[0 0 1 1 0]);disp('weights');
  "IW{3,2}(4,:)'" : Constant  Value=[-0.1653455096225807940957253094893530942499637603759765625;-1.081214726457761177158545251586474478244781494140625;-0.87422027289532888705281266084057278931140899658203125;0.450305492871755752570805952927912585437297821044921875;0.94119705017322896622999905957840383052825927734375;-0.230965046571925347596021538265631534159183502197265625;0.26598312393281398069433407727046869695186614990234375;-1.4602629612013602322662109145312570035457611083984375;0.533703661117485683718086875160224735736846923828125;0.58901819935871646549685465288348495960235595703125;-0.0670152521880752194416430711498833261430263519287109375;0.022246010270851886148069098680934985168278217315673828125;-0.39193717831722663103022341601899825036525726318359375;0.649176433325964641340988237061537802219390869140625;0.0500903295252175251306425707298330962657928466796875]
      mask Display: e = 0.06;c1 = [120 150 230]/255;c2 = ([120 150 230]+0)/383;c3 = ([120 150 230]+128)/383;patch([0 1 1 0],[0 0 1 1],c1);patch([0 1 1 1-e 1-e 0+e],[0 0 1 1-e 0+e 0+e],c2);patch([0 0 1 1-e 0+e 0+e],[0 1 1 1-e 1-e 0+e],c3);plot([0 1 1 0 0],[0 0 1 1 0]);disp('weights');
  "IW{3,2}(5,:)'" : Constant  Value=[-0.2045241583878916469263486987983924336731433868408203125;-0.125354316211277849735239442452439107000827789306640625;0.325213185635493673419915694466908462345600128173828125;0.96376666077028783075064666263642720878124237060546875;0.7338605835038318758734021685086190700531005859375;0.3512237265341091596582145939464680850505828857421875;0.92732155751110323382846445383620448410511016845703125;-0.95475943079519620670936319584143348038196563720703125;0.562058879210680206739425557316280901432037353515625;0.575612408601498426463649593642912805080413818359375;-0.9355246594441180008061564876697957515716552734375;0.8394894433523127919016815212671644985675811767578125;0.239565362120050029393070190053549595177173614501953125;-0.335353844366861719716865763984969817101955413818359375;-0.3483327424735016553114519410883076488971710205078125]
      mask Display: e = 0.06;c1 = [120 150 230]/255;c2 = ([120 150 230]+0)/383;c3 = ([120 150 230]+128)/383;patch([0 1 1 0],[0 0 1 1],c1);patch([0 1 1 1-e 1-e 0+e],[0 0 1 1-e 0+e 0+e],c2);patch([0 0 1 1-e 0+e 0+e],[0 1 1 1-e 1-e 0+e],c3);plot([0 1 1 0 0],[0 0 1 1 0]);disp('weights');
  "IW{3,2}(6,:)'" : Constant  Value=[-0.98670628691162221013399857838521711528301239013671875;0.1438209374104713333952787479574908502399921417236328125;0.11857811367303762450919890625300467945635318756103515625;0.483871831262136009588203933162731118500232696533203125;-0.8275309402730073315979097969830036163330078125;-0.032919301762808682310090802047852776013314723968505859375;-0.1498879768750767116358701969147659838199615478515625;0.1222687069894655420565499071017256937921047210693359375;-0.1801951938113963425092123316062497906386852264404296875;-0.267192962551895230038923045867704786360263824462890625;0.5956980791359203220025619884836487472057342529296875;-0.16539610149631422952865023034974001348018646240234375;1.089349735894892479137752161477692425251007080078125;-0.88664481566469210971348502425826154649257659912109375;0.0928988798061369802638864712207578122615814208984375]
      mask Display: e = 0.06;c1 = [120 150 230]/255;c2 = ([120 150 230]+0)/383;c3 = ([120 150 230]+128)/383;patch([0 1 1 0],[0 0 1 1],c1);patch([0 1 1 1-e 1-e 0+e],[0 0 1 1-e 0+e 0+e],c2);patch([0 0 1 1-e 0+e 0+e],[0 1 1 1-e 1-e 0+e],c3);plot([0 1 1 0 0],[0 0 1 1 0]);disp('weights');
  "IW{3,2}(7,:)'" : Constant  Value=[-0.40351205622447228194005219847895205020904541015625;-0.979326763313207226957501916331239044666290283203125;0.215731814525891518741218533250503242015838623046875;-0.735834088572874467359952177503146231174468994140625;-0.2671267673616022353400012434576638042926788330078125;-0.6963089497674668226778749158256687223911285400390625;0.3895043892358802661846084447461180388927459716796875;-0.14087108149629390396739836432971060276031494140625;-0.782364123453909154903840317274443805217742919921875;-0.631132664484693517437108312151394784450531005859375;-0.19522333460767615775921512977220118045806884765625;-0.3293773385895077954188536750734783709049224853515625;0.8714617455697608594533676296123303472995758056640625;0.3319744328222211660062157534412108361721038818359375;-0.20223849523360204472055556834675371646881103515625]
      mask Display: e = 0.06;c1 = [120 150 230]/255;c2 = ([120 150 230]+0)/383;c3 = ([120 150 230]+128)/383;patch([0 1 1 0],[0 0 1 1],c1);patch([0 1 1 1-e 1-e 0+e],[0 0 1 1-e 0+e 0+e],c2);patch([0 0 1 1-e 0+e 0+e],[0 1 1 1-e 1-e 0+e],c3);plot([0 1 1 0 0],[0 0 1 1 0]);disp('weights');
  "IW{3,2}(8,:)'" : Constant  Value=[-0.94373226930546394441989832557737827301025390625;-0.5833312606664506905218559040804393589496612548828125;0.0185919042278486212893540141521953046321868896484375;0.51203406407745843953449593755067326128482818603515625;-0.2616023913399636580123797102714888751506805419921875;0.249061080679932322912151221316889859735965728759765625;0.5171689688250296068616762568126432597637176513671875;-0.691726122903341344994032624526880681514739990234375;0.47255555345153510415912023745477199554443359375;-1.03717681399399896946533772279508411884307861328125;0.9910698100783397190838286405778490006923675537109375;-1.0418479970694107805684325285255908966064453125;0.5184078318095115545105500132194720208644866943359375;0.12010515088473018574521944401567452587187290191650390625;-0.16981322677390675579545131768099963665008544921875]
      mask Display: e = 0.06;c1 = [120 150 230]/255;c2 = ([120 150 230]+0)/383;c3 = ([120 150 230]+128)/383;patch([0 1 1 0],[0 0 1 1],c1);patch([0 1 1 1-e 1-e 0+e],[0 0 1 1-e 0+e 0+e],c2);patch([0 0 1 1-e 0+e 0+e],[0 1 1 1-e 1-e 0+e],c3);plot([0 1 1 0 0],[0 0 1 1 0]);disp('weights');
  "IW{3,2}(9,:)'" : Constant  Value=[0.010856284915405911561947505106218159198760986328125;0.3358322431472473557079183592577464878559112548828125;-0.7903735160530007686219278184580616652965545654296875;-0.7792930387153027549373973670299164950847625732421875;0.3700569453232185335167514494969509541988372802734375;-0.7987873552751569850016721829888410866260528564453125;-0.1347153477057989601206600127625279128551483154296875;0.2197143385804321003007544277352280914783477783203125;-0.7470002693413941852185189418378286063671112060546875;-0.8453063837746463971001276149763725697994232177734375;-0.195632029555030673151350129046477377414703369140625;-0.0948149168613519055526239753817208111286163330078125;-0.5190432063358307868128349582548253238201141357421875;0.0331164167025408406885844669886864721775054931640625;-0.63852447949041124530822344240732491016387939453125]
      mask Display: e = 0.06;c1 = [120 150 230]/255;c2 = ([120 150 230]+0)/383;c3 = ([120 150 230]+128)/383;patch([0 1 1 0],[0 0 1 1],c1);patch([0 1 1 1-e 1-e 0+e],[0 0 1 1-e 0+e 0+e],c2);patch([0 0 1 1-e 0+e 0+e],[0 1 1 1-e 1-e 0+e],c3);plot([0 1 1 0 0],[0 0 1 1 0]);disp('weights');
  Mux : Mux  Inputs=15
      mask Display: e = 0.06;c1 = [120 150 230]/255;c2 = ([120 150 230]+0)/383;c3 = ([120 150 230]+128)/383;patch([0 1 1 0],[0 0 1 1],c1);patch([0 1 1 1-e 1-e 0+e],[0 0 1 1-e 0+e 0+e],c2);patch([0 0 1 1-e 0+e 0+e],[0 1 1 1-e 1-e 0+e],c3);plot([0 1 1 0 0],[0 0 1 1 0]);disp('Mux');
  dotprod{1..15} (15 alike) : neural/Weight Functions/dotprod
  "lz{3,2}" : Outport
      mask Display: e = 0.06;c1 = [120 230 180]/255;c2 = ([120 230 180]+0)/(256+128);c3 = ([120 230 180]+128)/(256+128);patch([0 1 1 0],[0 0 1 1],c1);patch([0 1 1 1-e 1-e 0+e],[0 0 1 1-e 0+e 0+e],c2);patch([0 0 1 1-e 0+e 0+e],[0 1 1 1-e 1-e 0+e],c3);plot([0 1 1 0 0],[0 0 1 1 0]);
  wires:
  "IW{3,2}(1,:)'"/1 -> dotprod1/1
  "ad{3,2}"/1 -> dotprod1/2, dotprod2/2, dotprod3/2, dotprod4/2, dotprod5/2, dotprod6/2, dotprod7/2, dotprod8/2, dotprod9/2, dotprod10/2, dotprod11/2, dotprod12/2, dotprod13/2, dotprod14/2, dotprod15/2
  dotprod1/1 -> Mux/1
  "IW{3,2}(2,:)'"/1 -> dotprod2/1
  dotprod2/1 -> Mux/2
  "IW{3,2}(3,:)'"/1 -> dotprod3/1
  dotprod3/1 -> Mux/3
  "IW{3,2}(4,:)'"/1 -> dotprod4/1
  dotprod4/1 -> Mux/4
  "IW{3,2}(5,:)'"/1 -> dotprod5/1
  dotprod5/1 -> Mux/5
  "IW{3,2}(6,:)'"/1 -> dotprod6/1
  dotprod6/1 -> Mux/6
  "IW{3,2}(7,:)'"/1 -> dotprod7/1
  dotprod7/1 -> Mux/7
  "IW{3,2}(8,:)'"/1 -> dotprod8/1
  dotprod8/1 -> Mux/8
  "IW{3,2}(9,:)'"/1 -> dotprod9/1
  dotprod9/1 -> Mux/9
  "IW{3,2}(10,:)'"/1 -> dotprod10/1
  dotprod10/1 -> Mux/10
  "IW{3,2}(11,:)'"/1 -> dotprod11/1
  dotprod11/1 -> Mux/11
  "IW{3,2}(12,:)'"/1 -> dotprod12/1
  dotprod12/1 -> Mux/12
  "IW{3,2}(13,:)'"/1 -> dotprod13/1
  dotprod13/1 -> Mux/13
  "IW{3,2}(14,:)'"/1 -> dotprod14/1
  dotprod14/1 -> Mux/14
  "IW{3,2}(15,:)'"/1 -> dotprod15/1
  dotprod15/1 -> Mux/15
  Mux/1 -> "lz{3,2}"/1

== system Tactical_ACC_trainlm_3_15_Jan_5/Feed-Forward Neural Network/Layer 4/Delays 1 ==
  "p{4}" : Inport  PortDimensions=15
      mask Display: e = 0.06;c1 = [120 230 180]/255;c2 = ([120 230 180]+0)/(256+128);c3 = ([120 230 180]+128)/(256+128);patch([0 1 1 0],[0 0 1 1],c1);patch([0 1 1 1-e 1-e 0+e],[0 0 1 1-e 0+e 0+e],c2);patch([0 0 1 1-e 0+e 0+e],[0 1 1 1-e 1-e 0+e],c3);plot([0 1 1 0 0],[0 0 1 1 0]);
  mux : Mux  Inputs=1
      mask Display: e = 0.06;c1 = [120 150 230]/255;c2 = ([120 150 230]+0)/383;c3 = ([120 150 230]+128)/383;patch([0 1 1 0],[0 0 1 1],c1);patch([0 1 1 1-e 1-e 0+e],[0 0 1 1-e 0+e 0+e],c2);patch([0 0 1 1-e 0+e 0+e],[0 1 1 1-e 1-e 0+e],c3);plot([0 1 1 0 0],[0 0 1 1 0]);disp('Mux')
  "pd{4,3}" : Outport
      mask Display: e = 0.06;c1 = [120 230 180]/255;c2 = ([120 230 180]+0)/(256+128);c3 = ([120 230 180]+128)/(256+128);patch([0 1 1 0],[0 0 1 1],c1);patch([0 1 1 1-e 1-e 0+e],[0 0 1 1-e 0+e 0+e],c2);patch([0 0 1 1-e 0+e 0+e],[0 1 1 1-e 1-e 0+e],c3);plot([0 1 1 0 0],[0 0 1 1 0]);
  wires:
  "p{4}"/1 -> mux/1
  mux/1 -> "pd{4,3}"/1

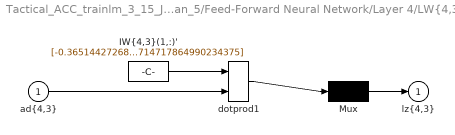
== system Tactical_ACC_trainlm_3_15_Jan_5/Feed-Forward Neural Network/Layer 4/LW{4,3} ==
  "ad{4,3}" : Inport  PortDimensions=15
      mask Display: e = 0.06;c1 = [120 230 180]/255;c2 = ([120 230 180]+0)/(256+128);c3 = ([120 230 180]+128)/(256+128);patch([0 1 1 0],[0 0 1 1],c1);patch([0 1 1 1-e 1-e 0+e],[0 0 1 1-e 0+e 0+e],c2);patch([0 0 1 1-e 0+e 0+e],[0 1 1 1-e 1-e 0+e],c3);plot([0 1 1 0 0],[0 0 1 1 0]);
  "IW{4,3}(1,:)'" : Constant  Value=[-0.365144272688300741691591611015610396862030029296875;0.6290795458013025420740405024844221770763397216796875;0.5781470298779165517544242902658879756927490234375;1.5199255259402597584283967080409638583660125732421875;-0.342205347540937399042348943112301640212535858154296875;0.82569404513210198359729474759660661220550537109375;0.9017888307562704763853389522409997880458831787109375;-0.90504561427777108217895829511689953505992889404296875;-0.879962360441048030423871750826947391033172607421875;1.2630287049350332750918823876418173313140869140625;0.26237746853802246249642848852090537548065185546875;-0.07904742004872937488624273782988893799483776092529296875;0.99400654321329540152873960323631763458251953125;-2.2230796200168470022617839276790618896484375;0.285608372544214839106047065797611139714717864990234375]
      mask Display: e = 0.06;c1 = [120 150 230]/255;c2 = ([120 150 230]+0)/383;c3 = ([120 150 230]+128)/383;patch([0 1 1 0],[0 0 1 1],c1);patch([0 1 1 1-e 1-e 0+e],[0 0 1 1-e 0+e 0+e],c2);patch([0 0 1 1-e 0+e 0+e],[0 1 1 1-e 1-e 0+e],c3);plot([0 1 1 0 0],[0 0 1 1 0]);disp('weights');
  Mux : Mux  Inputs=1
      mask Display: e = 0.06;c1 = [120 150 230]/255;c2 = ([120 150 230]+0)/383;c3 = ([120 150 230]+128)/383;patch([0 1 1 0],[0 0 1 1],c1);patch([0 1 1 1-e 1-e 0+e],[0 0 1 1-e 0+e 0+e],c2);patch([0 0 1 1-e 0+e 0+e],[0 1 1 1-e 1-e 0+e],c3);plot([0 1 1 0 0],[0 0 1 1 0]);disp('Mux');
  dotprod1 : neural/Weight Functions/dotprod
  "lz{4,3}" : Outport
      mask Display: e = 0.06;c1 = [120 230 180]/255;c2 = ([120 230 180]+0)/(256+128);c3 = ([120 230 180]+128)/(256+128);patch([0 1 1 0],[0 0 1 1],c1);patch([0 1 1 1-e 1-e 0+e],[0 0 1 1-e 0+e 0+e],c2);patch([0 0 1 1-e 0+e 0+e],[0 1 1 1-e 1-e 0+e],c3);plot([0 1 1 0 0],[0 0 1 1 0]);
  wires:
  "IW{4,3}(1,:)'"/1 -> dotprod1/1
  "ad{4,3}"/1 -> dotprod1/2
  dotprod1/1 -> Mux/1
  Mux/1 -> "lz{4,3}"/1
